simulink model "sampleModel240"  (R2021b)
settings: Solver=VariableStepAuto  StartTime=0.0  StopTime=10.0  RelTol=1e-3
undefined symbols (not defined in the file or in its folder): DiscIntNeverNeededParam, Newton, Raphson
libraries: simulink x11, slpidlib x4
settings Model: Creator=user  LastModifiedBy=user

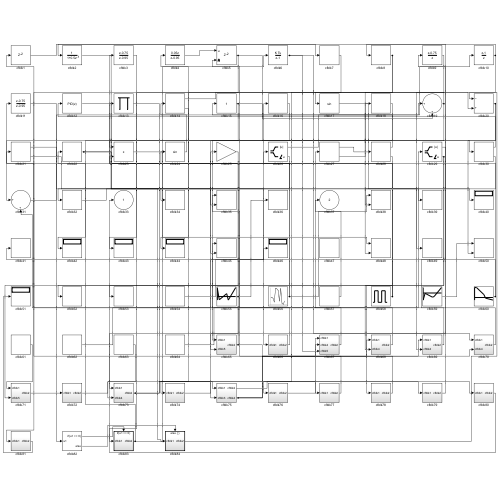
[thumbnail: Simulink's stored preview of the top-level diagram]
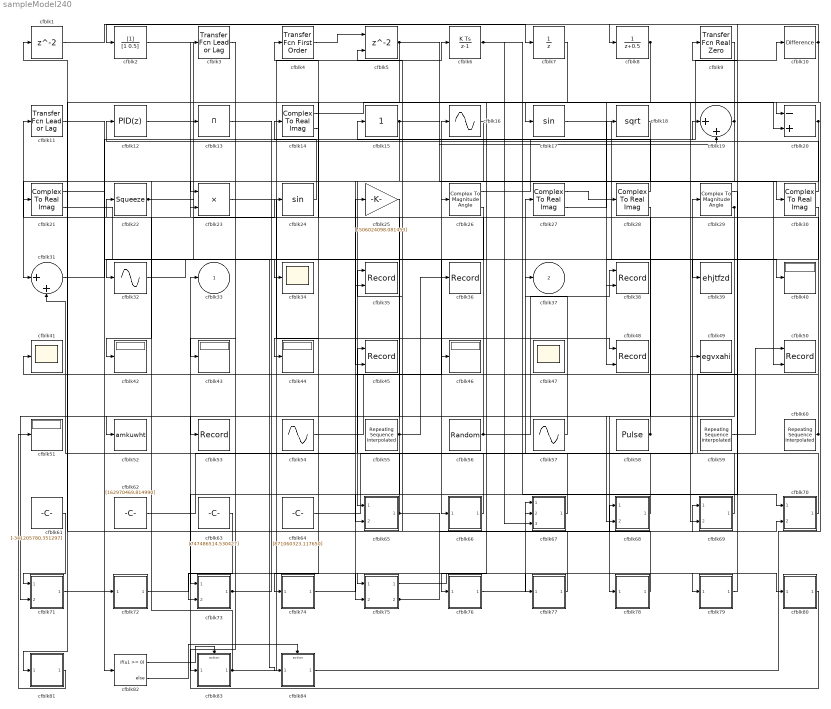
== system sampleModel240 ==
  cfblk1 : Delay  SampleTime=1
  cfblk10 : simulink/Discrete/Difference  ICPrevInput=0.0  OutMin=[]  OutMax=[]  OutDataTypeStr=Inherit: Inherit via back propagation  OutDataType=fixdt(1, 16)  OutScaling=2^-10  DoSatur=off
  cfblk11 : simulink/Discrete/Transfer Fcn Lead or Lag  PoleZ=0.95  ZeroZ=0.75  ICPrevOutput=0.0  ICPrevInput=0.0  DoSatur=off
      settings: SourceProductBaseCode=SL
  cfblk12 : slpidlib/PID Controller  Controller=PID  Form=Parallel  TimeDomain=Discrete-time  UseExternalTs=off  SampleTime=1  IntegratorMethod=Forward Euler  FilterMethod=Forward Euler  ControllerParametersSource=internal  P=1  I=1  D=0  UseFilter=on  N=100  TunerSelectOption=Transfer Function Based (PID Tuner App)  InitialConditionSource=internal  InitialConditionForIntegrator=0  InitialConditionForFilter=0  DifferentiatorICPrevScaledInput=0  ExternalReset=none  TrackingMode=off  Kt=1  LimitOutput=off  SatLimitsSource=internal  UpperSaturationLimit=inf  LowerSaturationLimit=-inf  LinearizeAsGain=off  AntiWindupMode=none  Kb=1  POutMin=[]  POutMax=[]  IOutMin=[]  IOutMax=[]  DOutMin=[]  DOutMax=[]  NOutMin=[]  NOutMax=[]  SumOutMin=[]  SumOutMax=[]  SaturationOutMin=[]  SaturationOutMax=[]  PParamMin=[]  PParamMax=[]  IParamMin=[]  IParamMax=[]  DParamMin=[]  DParamMax=[]  NParamMin=[]  NParamMax=[]  KbParamMin=[]  KbParamMax=[]  KtParamMin=[]  KtParamMax=[]  KbOutMin=[]  KbOutMax=[]  KtOutMin=[]  KtOutMax=[]  IntegratorOutMin=[]  IntegratorOutMax=[]  FilterOutMin=[]  FilterOutMax=[]  SumI1OutMin=[]  SumI1OutMax=[]  SumI2OutMin=[]  SumI2OutMax=[]  SumI3OutMin=[]  SumI3OutMax=[]  SumI4OutMin=[]  SumI4OutMax=[]  SumDOutMin=[]  SumDOutMax=[]  DifferentiatorOutMin=[]  DifferentiatorOutMax=[]  FilterDiffOutCoefMin=[]  FilterDiffOutCoefMax=[]  ReciprocalOutMin=[]  ReciprocalOutMax=[]  SumDenOutMin=[]  SumDenOutMax=[]  SumNumOutMin=[]  SumNumOutMax=[]  DivideOutMin=[]  DivideOutMax=[]  UdiffTsProdOutMin=[]  UdiffTsProdOutMax=[]  NTsProdOutMin=[]  NTsProdOutMax=[]  UintegralTsProdOutMin=[]  UintegralTsProdOutMax=[]  UngainTsProdOutMin=[]  UngainTsProdOutMax=[]  IntegratorContinuousStateAttributes=''  IntegratorStateMustResolveToSignalObject=off  IntegratorRTWStateStorageClass=Auto  FilterContinuousStateAttributes=''  FilterStateMustResolveToSignalObject=off  FilterRTWStateStorageClass=Auto  ParallelPVariant=InternalParameters  IdealPVariant=Disabled  IVariant=InternalParameters  DVariant=InternalParameters  IntegratorVariant=Discrete  SatVariant=Disabled  AWVariant=Passthrough  PCopyVariant=Disabled  TRVariant=Disabled  FdbkBlocksVariant=Forward  IdealPFdbkVariant=Disabled  SatFdbkVariant=Disabled  DerivativeFilterVariant=ForwardEulerFilter  NVariant=InternalParameters  NCopyVariant=Disabled  FilterICVariant=InternalICsFilter  IntegratorICVariant=InternalICs  ExternalResetVariant=Disabled  TRSumVariant=Passthrough  SumFdbkVariant=Disabled  SumVariant=Sum_PID  TsampFilterVariant=InternalTs  TsampNgainVariant=Passthrough  TsampIntegralVariant=Passthrough  ExternalSaturationOutDataTypeStr=Inherit: Same as second input
  cfblk13 : Product  Inputs=*
  cfblk{14,21,27..28,30} (5 alike) : ComplexToRealImag
  cfblk15 : simulink/Math Operations/Slider Gain  gain=1  low=0  high=2
  cfblk16 : Sin  TimeSource=Use external signal  SampleTime=0
  cfblk17 : Trigonometry
  cfblk18 : Sqrt  SaturateOnIntegerOverflow=on
  cfblk19 : Sum  Inputs=|++
  cfblk2 : DiscreteFilter  SampleTime=1
  cfblk20 : Sum  Inputs=-+
  cfblk22 : Squeeze
  cfblk23 : Product  Inputs=**
  cfblk24 : Trigonometry
  cfblk25 : Gain  Gain=[-506024098.081453]
  cfblk26 : ComplexToMagnitudeAngle
  cfblk29 : ComplexToMagnitudeAngle
  cfblk3 : simulink/Discrete/Transfer Fcn Lead or Lag  PoleZ=0.95  ZeroZ=0.75  ICPrevOutput=0.0  ICPrevInput=0.0  DoSatur=off
      settings: SourceProductBaseCode=SL
  cfblk31 : Sum  Inputs=|++
  cfblk32 : Sin  TimeSource=Use external signal  SampleTime=0
  cfblk34 : Scope
  cfblk35 : Record  FileSettingsInternal="{\"entries\":[{\"content\":{\"excelSettings\":{\"content\":{},\"type\":\"Streamout.ExcelSettings\"}},\"type\":\"Streamout.FileSettingStorage\",\"uuid\":\"784594ac-7453-4d0e-99dc-230d746005aa\"}],\"packageUris\":[\"http://schema.mathworks.com/mf0/streamout_blocks/R2020a\"],\"version\":\"1.0\"}"  Layout=[1 1]  SignalsInternal="{\"entries\":[{\"content\":{\"signals\":[{\"content\":{\"blockPath\":[\"sampleModel240/cfblk35\"],\"channel\":[],\"dimensions\":[1],\"domain\":\"sampleModel240/cfblk35\",\"lineColor\":\"#a2142f\",\"plots\":[1],\"port\":1,\"sid\":[\"\"],\"signalID\":9509,\"signalName\":\"cfblk78\"},\"type\":\"RecordBlkView.Signal\",\"uuid\":\"67d133b5-3512-448e-9778-6e57d9e23972\"},{\"content\":{\"blockPath\":[\"sampleModel240/cfblk35\"],\"channel\":[],\"dimensions\":[1],\"domain\":\"sampleModel240/cfblk35\",\"lineColor\":\"#139fff\",\"plots\":[1],\"port\":2,\"sid\":[\"\"],\"signalID\":9513,\"signalName\":\"cfblk11\"},\"type\":\"RecordBlkView.Signal\",\"uuid\":\"cb733c9c-883c-4945-886a-7784a95311ae\"}]},\"type\":\"RecordBlkView.InputSignals\",\"uuid\":\"c81b2700-d0a8-42b7-850e-26af2fe65ad5\"}],\"packageUris\":[\"http://schema.mathworks.com/mf0/streamout_blocks/R2020a\"],\"version\":\"1.0\"}"  VisualizationBindings="{\"xyplotplugin\":{\"info\":[{\"series\":[{\"bindingParametersList\":[{\"parameter\":\"X-Axis\",\"signalID\":9509,\"signalName\":\"cfblk78\"},{\"parameter\":\"Y-Axis\",\"signalID\":9513,\"signalName\":\"cfblk11\"}],\"seriesID\":32095}],\"subplotID\":1}]}}"  CompatibilityTag=XY
  cfblk36 : Record  FileSettingsInternal="{\"entries\":[{\"content\":{\"excelSettings\":{\"content\":{},\"type\":\"Streamout.ExcelSettings\"}},\"type\":\"Streamout.FileSettingStorage\",\"uuid\":\"b1a04026-dae7-46c6-8295-c1d018ed7cb2\"}],\"packageUris\":[\"http://schema.mathworks.com/mf0/streamout_blocks/R2020a\"],\"version\":\"1.0\"}"  SignalsInternal="{\"entries\":[{\"content\":{\"signals\":[{\"content\":{\"blockPath\":[\"sampleModel240/cfblk36\"],\"channel\":[],\"dimensions\":[1],\"domain\":\"sampleModel240/cfblk36\",\"lineColor\":\"#fe330a\",\"plots\":[1],\"port\":1,\"sid\":[\"\"],\"signalID\":9517,\"signalName\":\"cfblk55\"},\"type\":\"RecordBlkView.Signal\",\"uuid\":\"e81319b0-4fc9-46b2-b889-44dd591dc2c1\"}]},\"type\":\"RecordBlkView.InputSignals\",\"uuid\":\"d2d26a79-a2f7-4346-9dc2-1209bdb2fd03\"}],\"packageUris\":[\"http://schema.mathworks.com/mf0/streamout_blocks/R2020a\"],\"version\":\"1.0\"}"  VisualizationBindings="{\"sparklinesplugin\":{\"info\":[{\"bindingParametersList\":[],\"subplotID\":1}]}}"
  cfblk38 : Record  FileSettingsInternal="{\"entries\":[{\"content\":{\"excelSettings\":{\"content\":{},\"type\":\"Streamout.ExcelSettings\"}},\"type\":\"Streamout.FileSettingStorage\",\"uuid\":\"2b43e5d5-5da2-4669-81f9-69979c1bbe93\"}],\"packageUris\":[\"http://schema.mathworks.com/mf0/streamout_blocks/R2020a\"],\"version\":\"1.0\"}"  Layout=[1 1]  SignalsInternal="{\"entries\":[{\"content\":{\"signals\":[{\"content\":{\"blockPath\":[\"sampleModel240/cfblk38\"],\"channel\":[],\"dimensions\":[1],\"domain\":\"sampleModel240/cfblk38\",\"lineColor\":\"#a2142f\",\"plots\":[1],\"port\":1,\"sid\":[\"\"],\"signalID\":9521,\"signalName\":\"cfblk56\"},\"type\":\"RecordBlkView.Signal\",\"uuid\":\"72868b1f-4b0c-4be8-a2f7-40a7ef09af74\"},{\"content\":{\"blockPath\":[\"sampleModel240/cfblk38\"],\"channel\":[],\"dimensions\":[1],\"domain\":\"sampleModel240/cfblk38\",\"lineColor\":\"#139fff\",\"plots\":[1],\"port\":2,\"sid\":[\"\"],\"signalID\":9525,\"signalName\":\"cfblk30:2\"},\"type\":\"RecordBlkView.Signal\",\"uuid\":\"c76db0be-58e1-43fe-a83a-5ac3cfeabec3\"}]},\"type\":\"RecordBlkView.InputSignals\",\"uuid\":\"6d449aed-7e25-487a-9f87-ca08451d6c3a\"}],\"packageUris\":[\"http://schema.mathworks.com/mf0/streamout_blocks/R2020a\"],\"version\":\"1.0\"}"  VisualizationBindings="{\"xyplotplugin\":{\"info\":[{\"series\":[{\"bindingParametersList\":[{\"parameter\":\"X-Axis\",\"signalID\":9521,\"signalName\":\"cfblk56\"},{\"parameter\":\"Y-Axis\",\"signalID\":9525,\"signalName\":\"cfblk30:2\"}],\"seriesID\":59541}],\"subplotID\":1}]}}"  CompatibilityTag=XY
  cfblk39 : ToWorkspace  VariableName=ehjtfzd  SaveFormat=Timeseries  SampleTime=-1
  cfblk4 : simulink/Discrete/Transfer Fcn First Order  PoleZ=0.95  ICPrevOutput=0.0  DoSatur=off
  cfblk{40,42..44,46,51} (6 alike) : Display
  cfblk41 : Scope
  cfblk45 : Record  FileSettingsInternal="{\"entries\":[{\"content\":{\"excelSettings\":{\"content\":{},\"type\":\"Streamout.ExcelSettings\"}},\"type\":\"Streamout.FileSettingStorage\",\"uuid\":\"011ed913-79cb-4d04-904d-059d5477b360\"}],\"packageUris\":[\"http://schema.mathworks.com/mf0/streamout_blocks/R2020a\"],\"version\":\"1.0\"}"  Layout=[1 1]  SignalsInternal="{\"entries\":[{\"content\":{\"signals\":[{\"content\":{\"blockPath\":[\"sampleModel240/cfblk45\"],\"channel\":[],\"dimensions\":[1],\"domain\":\"sampleModel240/cfblk45\",\"lineColor\":\"#a2142f\",\"plots\":[1],\"port\":1,\"sid\":[\"\"],\"signalID\":9529,\"signalName\":\"cfblk67\"},\"type\":\"RecordBlkView.Signal\",\"uuid\":\"2900f96a-5edd-414d-b1fc-4191916f856c\"},{\"content\":{\"blockPath\":[\"sampleModel240/cfblk45\"],\"channel\":[],\"dimensions\":[1],\"domain\":\"sampleModel240/cfblk45\",\"lineColor\":\"#139fff\",\"plots\":[1],\"port\":2,\"sid\":[\"\"],\"signalID\":9533,\"signalName\":\"cfblk18\"},\"type\":\"RecordBlkView.Signal\",\"uuid\":\"83d649fc-fadd-439a-a8a7-d41cb33b9e8b\"}]},\"type\":\"RecordBlkView.InputSignals\",\"uuid\":\"9494aa0c-8dd6-4fcb-9a53-fd06893e11f2\"}],\"packageUris\":[\"http://schema.mathworks.com/mf0/streamout_blocks/R2020a\"],\"version\":\"1.0\"}"  VisualizationBindings="{\"xyplotplugin\":{\"info\":[{\"series\":[{\"bindingParametersList\":[{\"parameter\":\"X-Axis\",\"signalID\":9529,\"signalName\":\"cfblk67\"},{\"parameter\":\"Y-Axis\",\"signalID\":9533,\"signalName\":\"cfblk18\"}],\"seriesID\":51705}],\"subplotID\":1}]}}"  CompatibilityTag=XY
  cfblk47 : Scope
      settings: Floating=on
  cfblk48 : Record  FileSettingsInternal="{\"entries\":[{\"content\":{\"excelSettings\":{\"content\":{},\"type\":\"Streamout.ExcelSettings\"}},\"type\":\"Streamout.FileSettingStorage\",\"uuid\":\"3f33d199-868f-4f88-8702-0c4e5cfbf297\"}],\"packageUris\":[\"http://schema.mathworks.com/mf0/streamout_blocks/R2020a\"],\"version\":\"1.0\"}"  Layout=[1 1]  SignalsInternal="{\"entries\":[{\"content\":{\"signals\":[{\"content\":{\"blockPath\":[\"sampleModel240/cfblk48\"],\"channel\":[],\"dimensions\":[1],\"domain\":\"sampleModel240/cfblk48\",\"lineColor\":\"#a2142f\",\"plots\":[1],\"port\":1,\"sid\":[\"\"],\"signalID\":9537,\"signalName\":\"cfblk23\"},\"type\":\"RecordBlkView.Signal\",\"uuid\":\"ef2c7adb-1fb0-4c30-94cd-a61b1754e238\"},{\"content\":{\"blockPath\":[\"sampleModel240/cfblk48\"],\"channel\":[],\"dimensions\":[1],\"domain\":\"sampleModel240/cfblk48\",\"lineColor\":\"#139fff\",\"plots\":[1],\"port\":2,\"sid\":[\"\"],\"signalID\":9541,\"signalName\":\"cfblk8\"},\"type\":\"RecordBlkView.Signal\",\"uuid\":\"7ee245d3-5c2c-4c0d-a9a7-1766b601d128\"}]},\"type\":\"RecordBlkView.InputSignals\",\"uuid\":\"d6d367e3-47e7-4bb5-8610-e507c1deec50\"}],\"packageUris\":[\"http://schema.mathworks.com/mf0/streamout_blocks/R2020a\"],\"version\":\"1.0\"}"  VisualizationBindings="{\"xyplotplugin\":{\"info\":[{\"series\":[{\"bindingParametersList\":[{\"parameter\":\"X-Axis\",\"signalID\":9537,\"signalName\":\"cfblk23\"},{\"parameter\":\"Y-Axis\",\"signalID\":9541,\"signalName\":\"cfblk8\"}],\"seriesID\":9547}],\"subplotID\":1}]}}"  CompatibilityTag=XY
  cfblk49 : ToWorkspace  VariableName=egvxahi  SaveFormat=Timeseries  SampleTime=-1
  cfblk5 : Delay  ShowEnablePort=on  SampleTime=1
      settings: InputPortMap=u0,e6
  cfblk50 : Record  FileSettingsInternal="{\"entries\":[{\"content\":{\"excelSettings\":{\"content\":{},\"type\":\"Streamout.ExcelSettings\"}},\"type\":\"Streamout.FileSettingStorage\",\"uuid\":\"a7323de5-4913-44b3-ba6b-b7b4a20015af\"}],\"packageUris\":[\"http://schema.mathworks.com/mf0/streamout_blocks/R2020a\"],\"version\":\"1.0\"}"  Layout=[1 1]  SignalsInternal="{\"entries\":[{\"content\":{\"signals\":[{\"content\":{\"blockPath\":[\"sampleModel240/cfblk50\"],\"channel\":[],\"dimensions\":[1],\"domain\":\"sampleModel240/cfblk50\",\"lineColor\":\"#a2142f\",\"plots\":[1],\"port\":1,\"sid\":[\"\"],\"signalID\":9545,\"signalName\":\"cfblk59\"},\"type\":\"RecordBlkView.Signal\",\"uuid\":\"c6728527-33a3-402b-b809-e9ba282c6234\"},{\"content\":{\"blockPath\":[\"sampleModel240/cfblk50\"],\"channel\":[],\"dimensions\":[1],\"domain\":\"sampleModel240/cfblk50\",\"lineColor\":\"#139fff\",\"plots\":[1],\"port\":2,\"sid\":[\"\"],\"signalID\":9549,\"signalName\":\"cfblk20\"},\"type\":\"RecordBlkView.Signal\",\"uuid\":\"f80126da-2248-4c76-bb2b-053e64c3d372\"}]},\"type\":\"RecordBlkView.InputSignals\",\"uuid\":\"537812bb-574c-401c-a38e-823000144505\"}],\"packageUris\":[\"http://schema.mathworks.com/mf0/streamout_blocks/R2020a\"],\"version\":\"1.0\"}"  VisualizationBindings="{\"xyplotplugin\":{\"info\":[{\"series\":[{\"bindingParametersList\":[{\"parameter\":\"X-Axis\",\"signalID\":9545,\"signalName\":\"cfblk59\"},{\"parameter\":\"Y-Axis\",\"signalID\":9549,\"signalName\":\"cfblk20\"}],\"seriesID\":24204}],\"subplotID\":1}]}}"  CompatibilityTag=XY
  cfblk52 : ToWorkspace  VariableName=amkuwht  SaveFormat=Timeseries  SampleTime=-1
  cfblk53 : Record  FileSettingsInternal="{\"entries\":[{\"content\":{\"excelSettings\":{\"content\":{},\"type\":\"Streamout.ExcelSettings\"}},\"type\":\"Streamout.FileSettingStorage\",\"uuid\":\"062d2fcb-1db7-4794-8512-aa17b3a50389\"}],\"packageUris\":[\"http://schema.mathworks.com/mf0/streamout_blocks/R2020a\"],\"version\":\"1.0\"}"  SignalsInternal="{\"entries\":[{\"content\":{\"signals\":[{\"content\":{\"blockPath\":[\"sampleModel240/cfblk53\"],\"channel\":[],\"dimensions\":[1],\"domain\":\"sampleModel240/cfblk53\",\"lineColor\":\"#139fff\",\"plots\":[1],\"port\":1,\"sid\":[\"\"],\"signalID\":9553,\"signalName\":\"cfblk5\"},\"type\":\"RecordBlkView.Signal\",\"uuid\":\"004bb81a-6ea3-4587-b6bd-6712f3703243\"}]},\"type\":\"RecordBlkView.InputSignals\",\"uuid\":\"4f08d72a-b7cb-43bf-9134-c95f940a5c70\"}],\"packageUris\":[\"http://schema.mathworks.com/mf0/streamout_blocks/R2020a\"],\"version\":\"1.0\"}"  VisualizationBindings="{\"sparklinesplugin\":{\"info\":[{\"bindingParametersList\":[],\"subplotID\":1}]}}"
  cfblk54 : Sin  Amplitude=[927282513.188277]  Bias=[-745493718.771142]  SampleTime=0
  cfblk55 : simulink/Sources/Repeating Sequence Interpolated  OutValues=[757544215.990310, -282071434.589029, 262873848.324371, -311269752.017773, 843048073.550432]  TimeValues=[0 0.1 0.5 0.6 1].'  LookUpMeth=Use Input Nearest  tsamp=0.01  OutMin=[]  OutMax=[]  OutDataTypeStr=double  OutputDataTypeScalingMode=double  OutDataType=fixdt(0,8)  OutScaling=2^-10
  cfblk56 : RandomNumber  Mean=[-10045.091864]  Variance=[72480.359942]  Seed=[426711266.000000]  SampleTime=0.1
  cfblk57 : Sin  Amplitude=[314477199.179577]  Bias=[-113427137.959207]  SampleTime=0
  cfblk58 : DiscretePulseGenerator  PulseType=Time based  Amplitude=[121664850.347592]  Period=[59251250.117236]  PulseWidth=5  PhaseDelay=[3.000000]
  cfblk59 : simulink/Sources/Repeating Sequence Interpolated  OutValues=[-995730294.606779, -23875285.976552, -567680596.972897, -484368832.556859, 819766545.228171]  TimeValues=[0 0.1 0.5 0.6 1].'  LookUpMeth=Use Input Above  tsamp=0.01  OutMin=[]  OutMax=[]  OutDataTypeStr=double  OutputDataTypeScalingMode=double  OutDataType=fixdt(0,8)  OutScaling=2^-10
  cfblk6 : DiscreteIntegrator  ICPrevOutput=DiscIntNeverNeededParam  ICPrevScaledInput=DiscIntNeverNeededParam
  cfblk60 : simulink/Sources/Repeating Sequence Interpolated  OutValues=[884652968.497208, 878168725.746222, 262963678.617603, -60188493.029042, -217965531.630262]  TimeValues=[0 0.1 0.5 0.6 1].'  LookUpMeth=Use Input Nearest  tsamp=0.01  OutMin=[]  OutMax=[]  OutDataTypeStr=double  OutputDataTypeScalingMode=double  OutDataType=fixdt(0,8)  OutScaling=2^-10
  cfblk61 : Constant  Value=[-341205780.351297]  SampleTime=1
  cfblk62 : Constant  Value=[162970469.814990]  SampleTime=1
  cfblk63 : Constant  Value=[747486514.530427]  SampleTime=1
  cfblk64 : Constant  Value=[871060323.117650]  SampleTime=1
  cfblk65 : Subsystem
  cfblk66 : Subsystem
  cfblk67 : Subsystem
  cfblk68 : Subsystem
  cfblk69 : Subsystem
  cfblk7 : UnitDelay  HasFrameUpgradeWarning=on
  cfblk70 : Subsystem
  cfblk71 : Subsystem
  cfblk72 : Subsystem
  cfblk73 : Subsystem
  cfblk74 : Subsystem
  cfblk75 : Subsystem
  cfblk76 : Subsystem
  cfblk77 : Subsystem
  cfblk78 : Subsystem
  cfblk79 : Subsystem
  cfblk8 : DiscreteTransferFcn  SampleTime=1
  cfblk80 : Subsystem
  cfblk81 : Subsystem
  cfblk82 : If  IfExpression=u1 >= 0  SampleTime=1
  cfblk83 : Subsystem  TreatAsAtomicUnit=on
  cfblk84 : Subsystem  TreatAsAtomicUnit=on
  cfblk9 : simulink/Discrete/Transfer Fcn Real Zero  ZeroZ=0.75  ICPrevInput=0.0  DoSatur=off
      settings: SourceProductBaseCode=SL
  cfblk33 : Outport
  cfblk37 : Outport  Port=2
  wires:
  cfblk58/1 -> cfblk11/1, cfblk52/1, cfblk23/2
  cfblk83/1(cfblk2) -> cfblk6/1, cfblk22/1
  cfblk64/1 -> cfblk29/1
  cfblk75/1(cfblk2) -> cfblk79/1(cfblk1)
  cfblk59/1 -> cfblk50/1
  cfblk24/1 -> cfblk14/1
  cfblk80/1(cfblk2) -> cfblk33/1
  cfblk8/1 -> cfblk74/1(cfblk1), cfblk48/2
  cfblk15/1 -> cfblk31/1, cfblk30/1
  cfblk79/1(cfblk2) -> cfblk2/1
  cfblk26/1 -> cfblk10/1
  cfblk32/1 -> cfblk84/1(cfblk1)
  cfblk16/1 -> cfblk65/1(cfblk1)
  cfblk67/1(cfblk2) -> cfblk45/1
  cfblk1/1 -> cfblk7/1
  cfblk26/2 -> cfblk32/1
  cfblk17/1 -> cfblk39/1
  cfblk18/1 -> cfblk45/2
  cfblk29/1 -> cfblk65/2(cfblk5)
  cfblk27/1 -> cfblk28/1
  cfblk54/1 -> cfblk16/1
  cfblk12/1 -> cfblk66/1(cfblk1)
  cfblk4/1 -> cfblk5/1
  cfblk70/1(cfblk2) -> cfblk9/1
  cfblk61/1 -> cfblk71/1(cfblk1)
  cfblk10/1 -> cfblk8/1, cfblk69/2(cfblk4)
  cfblk60/1 -> cfblk41/1, cfblk13/1
  cfblk55/1 -> cfblk73/1(cfblk1), cfblk3/1, cfblk36/1
  cfblk2/1 -> cfblk40/1
  cfblk20/1 -> cfblk42/1, cfblk50/2
  cfblk27/2 -> cfblk18/1
  cfblk69/1(cfblk2) -> cfblk5/2
  cfblk23/1 -> cfblk48/1
  cfblk62/1 -> cfblk25/1
  cfblk6/1 -> cfblk70/1(cfblk1), cfblk67/3(cfblk5)
  cfblk5/1 -> cfblk53/1, cfblk19/2
  cfblk7/1 -> cfblk81/1(cfblk1)
  cfblk63/1 -> cfblk73/2(cfblk4)
  cfblk68/1(cfblk2) -> cfblk27/1
  cfblk9/1 -> cfblk76/1(cfblk1)
  cfblk84/1(cfblk2) -> cfblk20/1
  cfblk22/1 -> cfblk34/1, cfblk24/1
  cfblk28/1 -> cfblk15/1
  cfblk19/1 -> cfblk17/1, cfblk23/1
  cfblk73/1(cfblk2) -> cfblk75/1(cfblk1), cfblk77/1(cfblk1)
  cfblk3/1 -> cfblk43/1
  cfblk56/1 -> cfblk38/1, cfblk26/1, cfblk4/1
  cfblk21/1 -> cfblk82/1
  cfblk30/1 -> cfblk12/1
  cfblk78/1(cfblk2) -> cfblk35/1
  cfblk57/1 -> cfblk37/1
  cfblk21/2 -> cfblk49/1
  cfblk31/1 -> cfblk19/1
  cfblk30/2 -> cfblk38/2
  cfblk71/1(cfblk2) -> cfblk72/1(cfblk1)
  cfblk66/1(cfblk2) -> cfblk31/2
  cfblk25/1 -> cfblk83/1(cfblk1)
  cfblk81/1(cfblk2) -> cfblk51/1
  cfblk28/2 -> cfblk71/2(cfblk5)
  cfblk14/1 -> cfblk20/2
  cfblk13/1 -> cfblk75/2(cfblk3)
  cfblk65/1(cfblk2) -> cfblk1/1, cfblk70/2(cfblk4)
  cfblk29/2 -> cfblk78/1(cfblk1), cfblk68/2(cfblk4)
  cfblk11/1 -> cfblk35/2
  cfblk72/1(cfblk2) -> cfblk80/1(cfblk1)
  cfblk14/2 -> cfblk44/1
  cfblk74/1(cfblk2) -> cfblk46/1
  cfblk77/1(cfblk2) -> cfblk21/1
  cfblk75/2(cfblk4) -> cfblk68/1(cfblk1), cfblk69/1(cfblk1), cfblk67/2(cfblk4)
  cfblk76/1(cfblk2) -> cfblk67/1(cfblk1)
  cfblk82/1 -> cfblk83/Action
  cfblk82/2 -> cfblk84/Action

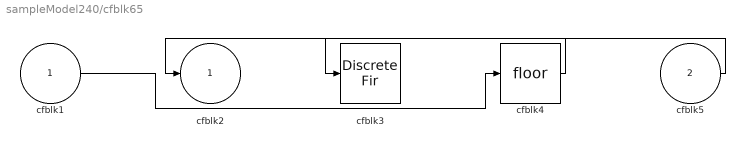
== system sampleModel240/cfblk65 ==
  cfblk1 : Inport
  cfblk5 : Inport  Port=2
  cfblk3 : DiscreteFir  SampleTime=1
  cfblk4 : Rounding
  cfblk2 : Outport
  wires:
  cfblk4/1 -> cfblk2/1
  cfblk1/1 -> cfblk4/1
  cfblk5/1 -> cfblk3/1

== system sampleModel240/cfblk66 ==
  cfblk1 : Inport
  cfblk3 : simulink/Discrete/Transfer Fcn Lead or Lag  PoleZ=0.95  ZeroZ=0.75  ICPrevOutput=0.0  ICPrevInput=0.0  DoSatur=off
      settings: SourceProductBaseCode=SL
  cfblk2 : Outport
  wires:
  cfblk3/1 -> cfblk2/1
  cfblk1/1 -> cfblk3/1

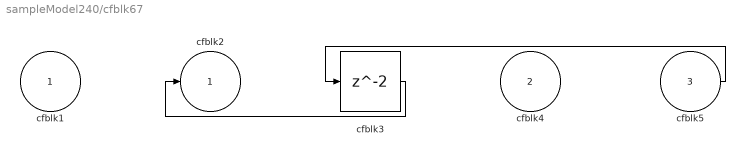
== system sampleModel240/cfblk67 ==
  cfblk1 : Inport
  cfblk4 : Inport  Port=2
  cfblk5 : Inport  Port=3
  cfblk3 : Delay  SampleTime=1
  cfblk2 : Outport
  wires:
  cfblk5/1 -> cfblk3/1
  cfblk3/1 -> cfblk2/1

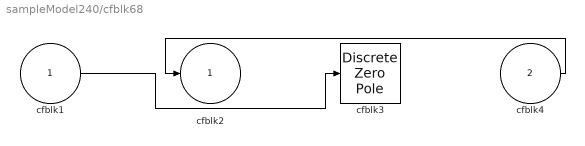
== system sampleModel240/cfblk68 ==
  cfblk1 : Inport
  cfblk4 : Inport  Port=2
  cfblk3 : DiscreteZeroPole  Poles=[0 0.5]  Gain=1
  cfblk2 : Outport
  wires:
  cfblk4/1 -> cfblk2/1
  cfblk1/1 -> cfblk3/1

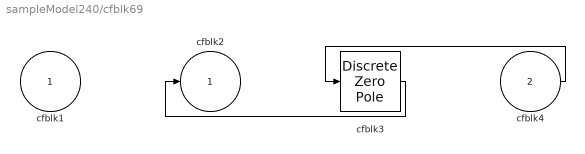
== system sampleModel240/cfblk69 ==
  cfblk1 : Inport
  cfblk4 : Inport  Port=2
  cfblk3 : DiscreteZeroPole  Poles=[0 0.5]  Gain=1
  cfblk2 : Outport
  wires:
  cfblk4/1 -> cfblk3/1
  cfblk3/1 -> cfblk2/1

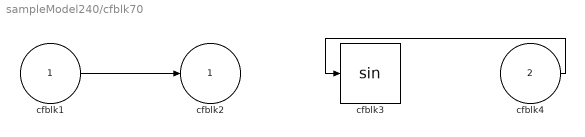
== system sampleModel240/cfblk70 ==
  cfblk1 : Inport
  cfblk4 : Inport  Port=2
  cfblk3 : Trigonometry
  cfblk2 : Outport
  wires:
  cfblk4/1 -> cfblk3/1
  cfblk1/1 -> cfblk2/1

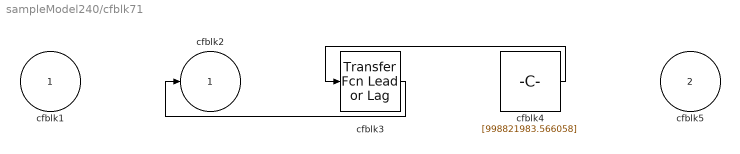
== system sampleModel240/cfblk71 ==
  cfblk1 : Inport
  cfblk5 : Inport  Port=2
  cfblk3 : simulink/Discrete/Transfer Fcn Lead or Lag  PoleZ=0.95  ZeroZ=0.75  ICPrevOutput=0.0  ICPrevInput=0.0  DoSatur=off
      settings: SourceProductBaseCode=SL
  cfblk4 : Constant  Value=[998821983.566058]  SampleTime=1
  cfblk2 : Outport
  wires:
  cfblk4/1 -> cfblk3/1
  cfblk3/1 -> cfblk2/1

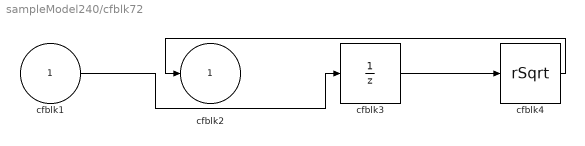
== system sampleModel240/cfblk72 ==
  cfblk1 : Inport
  cfblk3 : UnitDelay  HasFrameUpgradeWarning=on
  cfblk4 : Sqrt  Operator=rSqrt  AlgorithmType=Newton-Raphson  SaturateOnIntegerOverflow=on
  cfblk2 : Outport
  wires:
  cfblk4/1 -> cfblk2/1
  cfblk1/1 -> cfblk3/1
  cfblk3/1 -> cfblk4/1

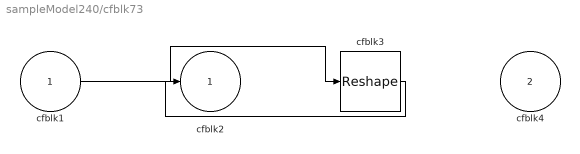
== system sampleModel240/cfblk73 ==
  cfblk1 : Inport
  cfblk4 : Inport  Port=2
  cfblk3 : Reshape
  cfblk2 : Outport
  wires:
  cfblk1/1 -> cfblk3/1
  cfblk3/1 -> cfblk2/1

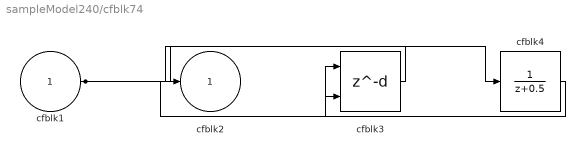
== system sampleModel240/cfblk74 ==
  cfblk1 : Inport
  cfblk3 : Delay  DelayLengthSource=Input port  SampleTime=1
      settings: InputPortMap=u0,p1
  cfblk4 : DiscreteTransferFcn  SampleTime=1
  cfblk2 : Outport
  wires:
  cfblk1/1 -> cfblk4/1, cfblk3/2
  cfblk4/1 -> cfblk3/1
  cfblk3/1 -> cfblk2/1

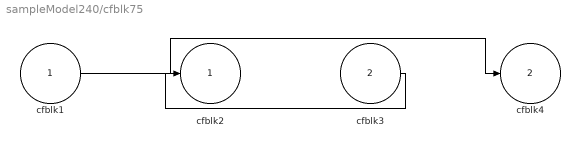
== system sampleModel240/cfblk75 ==
  cfblk1 : Inport
  cfblk3 : Inport  Port=2
  cfblk2 : Outport
  cfblk4 : Outport  Port=2
  wires:
  cfblk1/1 -> cfblk4/1
  cfblk3/1 -> cfblk2/1

== system sampleModel240/cfblk76 ==
  cfblk1 : Inport
  cfblk3 : Product  Inputs=**
  cfblk2 : Outport
  wires:
  cfblk1/1 -> cfblk3/1, cfblk3/2
  cfblk3/1 -> cfblk2/1

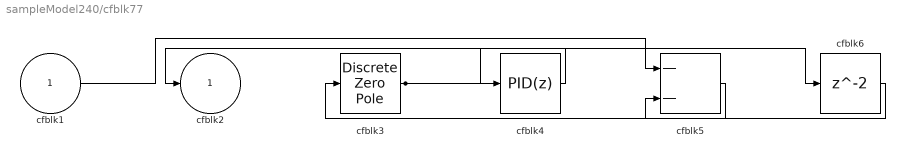
== system sampleModel240/cfblk77 ==
  cfblk1 : Inport
  cfblk3 : DiscreteZeroPole  Poles=[0 0.5]  Gain=1
  cfblk4 : slpidlib/PID Controller  Controller=PID  Form=Parallel  TimeDomain=Discrete-time  UseExternalTs=off  SampleTime=1  IntegratorMethod=Forward Euler  FilterMethod=Forward Euler  ControllerParametersSource=internal  P=1  I=1  D=0  UseFilter=on  N=100  TunerSelectOption=Transfer Function Based (PID Tuner App)  InitialConditionSource=internal  InitialConditionForIntegrator=0  InitialConditionForFilter=0  DifferentiatorICPrevScaledInput=0  ExternalReset=none  TrackingMode=off  Kt=1  LimitOutput=off  SatLimitsSource=internal  UpperSaturationLimit=inf  LowerSaturationLimit=-inf  LinearizeAsGain=off  AntiWindupMode=none  Kb=1  POutMin=[]  POutMax=[]  IOutMin=[]  IOutMax=[]  DOutMin=[]  DOutMax=[]  NOutMin=[]  NOutMax=[]  SumOutMin=[]  SumOutMax=[]  SaturationOutMin=[]  SaturationOutMax=[]  PParamMin=[]  PParamMax=[]  IParamMin=[]  IParamMax=[]  DParamMin=[]  DParamMax=[]  NParamMin=[]  NParamMax=[]  KbParamMin=[]  KbParamMax=[]  KtParamMin=[]  KtParamMax=[]  KbOutMin=[]  KbOutMax=[]  KtOutMin=[]  KtOutMax=[]  IntegratorOutMin=[]  IntegratorOutMax=[]  FilterOutMin=[]  FilterOutMax=[]  SumI1OutMin=[]  SumI1OutMax=[]  SumI2OutMin=[]  SumI2OutMax=[]  SumI3OutMin=[]  SumI3OutMax=[]  SumI4OutMin=[]  SumI4OutMax=[]  SumDOutMin=[]  SumDOutMax=[]  DifferentiatorOutMin=[]  DifferentiatorOutMax=[]  FilterDiffOutCoefMin=[]  FilterDiffOutCoefMax=[]  ReciprocalOutMin=[]  ReciprocalOutMax=[]  SumDenOutMin=[]  SumDenOutMax=[]  SumNumOutMin=[]  SumNumOutMax=[]  DivideOutMin=[]  DivideOutMax=[]  UdiffTsProdOutMin=[]  UdiffTsProdOutMax=[]  NTsProdOutMin=[]  NTsProdOutMax=[]  UintegralTsProdOutMin=[]  UintegralTsProdOutMax=[]  UngainTsProdOutMin=[]  UngainTsProdOutMax=[]  IntegratorContinuousStateAttributes=''  IntegratorStateMustResolveToSignalObject=off  IntegratorRTWStateStorageClass=Auto  FilterContinuousStateAttributes=''  FilterStateMustResolveToSignalObject=off  FilterRTWStateStorageClass=Auto  ParallelPVariant=InternalParameters  IdealPVariant=Disabled  IVariant=InternalParameters  DVariant=InternalParameters  IntegratorVariant=Discrete  SatVariant=Disabled  AWVariant=Passthrough  PCopyVariant=Disabled  TRVariant=Disabled  FdbkBlocksVariant=Forward  IdealPFdbkVariant=Disabled  SatFdbkVariant=Disabled  DerivativeFilterVariant=ForwardEulerFilter  NVariant=InternalParameters  NCopyVariant=Disabled  FilterICVariant=InternalICsFilter  IntegratorICVariant=InternalICs  ExternalResetVariant=Disabled  TRSumVariant=Passthrough  SumFdbkVariant=Disabled  SumVariant=Sum_PID  TsampFilterVariant=InternalTs  TsampNgainVariant=Passthrough  TsampIntegralVariant=Passthrough  ExternalSaturationOutDataTypeStr=Inherit: Same as second input
  cfblk5 : Sum  Inputs=--
  cfblk6 : Delay  SampleTime=1
  cfblk2 : Outport
  wires:
  cfblk4/1 -> cfblk2/1
  cfblk3/1 -> cfblk4/1, cfblk6/1
  cfblk1/1 -> cfblk5/1
  cfblk5/1 -> cfblk3/1
  cfblk6/1 -> cfblk5/2

== system sampleModel240/cfblk78 ==
  cfblk1 : Inport
  cfblk3 : DiscreteFir  SampleTime=1
  cfblk2 : Outport
  wires:
  cfblk1/1 -> cfblk2/1, cfblk3/1

== system sampleModel240/cfblk79 ==
  cfblk1 : Inport
  cfblk3 : Delay  DelayLengthSource=Input port  SampleTime=1
      settings: InputPortMap=u0,p1
  cfblk2 : Outport
  wires:
  cfblk1/1 -> cfblk2/1, cfblk3/1, cfblk3/2

== system sampleModel240/cfblk80 ==
  cfblk1 : Inport
  cfblk3 : slpidlib/PID Controller (2DOF)  Controller=PID  Form=Parallel  TimeDomain=Discrete-time  UseExternalTs=off  SampleTime=1  IntegratorMethod=Forward Euler  FilterMethod=Forward Euler  ControllerParametersSource=internal  P=1  I=1  D=0  UseFilter=on  N=100  b=1  c=1  TunerSelectOption=Transfer Function Based (PID Tuner App)  InitialConditionSource=internal  InitialConditionForIntegrator=0  InitialConditionForFilter=0  DifferentiatorICPrevScaledInput=0  ExternalReset=none  TrackingMode=off  Kt=1  LimitOutput=off  SatLimitsSource=internal  UpperSaturationLimit=inf  LowerSaturationLimit=-inf  LinearizeAsGain=off  AntiWindupMode=none  Kb=1  POutMin=[]  POutMax=[]  IOutMin=[]  IOutMax=[]  DOutMin=[]  DOutMax=[]  NOutMin=[]  NOutMax=[]  bOutMin=[]  bOutMax=[]  cOutMin=[]  cOutMax=[]  SumOutMin=[]  SumOutMax=[]  SaturationOutMin=[]  SaturationOutMax=[]  PParamMin=[]  PParamMax=[]  IParamMin=[]  IParamMax=[]  DParamMin=[]  DParamMax=[]  NParamMin=[]  NParamMax=[]  bParamMin=[]  bParamMax=[]  cParamMin=[]  cParamMax=[]  KbParamMin=[]  KbParamMax=[]  KtParamMin=[]  KtParamMax=[]  KbOutMin=[]  KbOutMax=[]  KtOutMin=[]  KtOutMax=[]  IntegratorOutMin=[]  IntegratorOutMax=[]  FilterOutMin=[]  FilterOutMax=[]  SumI1OutMin=[]  SumI1OutMax=[]  SumI2OutMin=[]  SumI2OutMax=[]  SumI3OutMin=[]  SumI3OutMax=[]  SumI4OutMin=[]  SumI4OutMax=[]  SumDOutMin=[]  SumDOutMax=[]  Sum1OutMin=[]  Sum1OutMax=[]  Sum2OutMin=[]  Sum2OutMax=[]  Sum3OutMin=[]  Sum3OutMax=[]  DifferentiatorOutMin=[]  DifferentiatorOutMax=[]  FilterDiffOutCoefMin=[]  FilterDiffOutCoefMax=[]  ReciprocalOutMin=[]  ReciprocalOutMax=[]  SumDenOutMin=[]  SumDenOutMax=[]  SumNumOutMin=[]  SumNumOutMax=[]  DivideOutMin=[]  DivideOutMax=[]  UdiffTsProdOutMin=[]  UdiffTsProdOutMax=[]  NTsProdOutMin=[]  NTsProdOutMax=[]  UintegralTsProdOutMin=[]  UintegralTsProdOutMax=[]  UngainTsProdOutMin=[]  UngainTsProdOutMax=[]  IntegratorContinuousStateAttributes=''  IntegratorStateMustResolveToSignalObject=off  IntegratorRTWStateStorageClass=Auto  FilterContinuousStateAttributes=''  FilterStateMustResolveToSignalObject=off  FilterRTWStateStorageClass=Auto  ParallelPVariant=InternalParameters  IdealPVariant=Disabled  IVariant=InternalParameters  DVariant=InternalParameters  bVariant=InternalParameters  cVariant=InternalParameters  IntegratorVariant=Discrete  SatVariant=Disabled  AWVariant=Passthrough  PCopyVariant=Disabled  TRVariant=Disabled  FdbkBlocksVariant=Forward  IdealPFdbkVariant=Disabled  SatFdbkVariant=Disabled  DerivativeFilterVariant=ForwardEulerFilter  NVariant=InternalParameters  NCopyVariant=Disabled  FilterICVariant=InternalICsFilter  IntegratorICVariant=InternalICs  ExternalResetVariant=Disabled  TRSumVariant=Passthrough  SumFdbkVariant=Disabled  SumVariant=Sum_PID  TsampFilterVariant=InternalTs  TsampNgainVariant=Passthrough  TsampIntegralVariant=Passthrough  ExternalSaturationOutDataTypeStr=Inherit: Same as second input
      settings: SourceProductBaseCode=SL
  cfblk2 : Outport
  wires:
  cfblk1/1 -> cfblk3/1, cfblk3/2
  cfblk3/1 -> cfblk2/1

== system sampleModel240/cfblk81 ==
  cfblk1 : Inport
  cfblk3 : Constant  Value=[-203881698.198706]  SampleTime=1
  cfblk2 : Outport
  wires:
  cfblk3/1 -> cfblk2/1

== system sampleModel240/cfblk83 ==
  cfblk1 : Inport
  Action Port : ActionPort  ActionPortLabel=if(u1 >= 0)
  cfblk3 : slpidlib/PID Controller  Controller=PID  Form=Parallel  TimeDomain=Discrete-time  UseExternalTs=off  SampleTime=-1  IntegratorMethod=Forward Euler  FilterMethod=Forward Euler  ControllerParametersSource=internal  P=1  I=1  D=0  UseFilter=on  N=100  TunerSelectOption=Transfer Function Based (PID Tuner App)  InitialConditionSource=internal  InitialConditionForIntegrator=0  InitialConditionForFilter=0  DifferentiatorICPrevScaledInput=0  ExternalReset=none  TrackingMode=off  Kt=1  LimitOutput=off  SatLimitsSource=internal  UpperSaturationLimit=inf  LowerSaturationLimit=-inf  LinearizeAsGain=off  AntiWindupMode=none  Kb=1  POutMin=[]  POutMax=[]  IOutMin=[]  IOutMax=[]  DOutMin=[]  DOutMax=[]  NOutMin=[]  NOutMax=[]  SumOutMin=[]  SumOutMax=[]  SaturationOutMin=[]  SaturationOutMax=[]  PParamMin=[]  PParamMax=[]  IParamMin=[]  IParamMax=[]  DParamMin=[]  DParamMax=[]  NParamMin=[]  NParamMax=[]  KbParamMin=[]  KbParamMax=[]  KtParamMin=[]  KtParamMax=[]  KbOutMin=[]  KbOutMax=[]  KtOutMin=[]  KtOutMax=[]  IntegratorOutMin=[]  IntegratorOutMax=[]  FilterOutMin=[]  FilterOutMax=[]  SumI1OutMin=[]  SumI1OutMax=[]  SumI2OutMin=[]  SumI2OutMax=[]  SumI3OutMin=[]  SumI3OutMax=[]  SumI4OutMin=[]  SumI4OutMax=[]  SumDOutMin=[]  SumDOutMax=[]  DifferentiatorOutMin=[]  DifferentiatorOutMax=[]  FilterDiffOutCoefMin=[]  FilterDiffOutCoefMax=[]  ReciprocalOutMin=[]  ReciprocalOutMax=[]  SumDenOutMin=[]  SumDenOutMax=[]  SumNumOutMin=[]  SumNumOutMax=[]  DivideOutMin=[]  DivideOutMax=[]  UdiffTsProdOutMin=[]  UdiffTsProdOutMax=[]  NTsProdOutMin=[]  NTsProdOutMax=[]  UintegralTsProdOutMin=[]  UintegralTsProdOutMax=[]  UngainTsProdOutMin=[]  UngainTsProdOutMax=[]  IntegratorContinuousStateAttributes=''  IntegratorStateMustResolveToSignalObject=off  IntegratorRTWStateStorageClass=Auto  FilterContinuousStateAttributes=''  FilterStateMustResolveToSignalObject=off  FilterRTWStateStorageClass=Auto  ParallelPVariant=InternalParameters  IdealPVariant=Disabled  IVariant=InternalParameters  DVariant=InternalParameters  IntegratorVariant=Discrete  SatVariant=Disabled  AWVariant=Passthrough  PCopyVariant=Disabled  TRVariant=Disabled  FdbkBlocksVariant=Forward  IdealPFdbkVariant=Disabled  SatFdbkVariant=Disabled  DerivativeFilterVariant=ForwardEulerFilter  NVariant=InternalParameters  NCopyVariant=Disabled  FilterICVariant=InternalICsFilter  IntegratorICVariant=InternalICs  ExternalResetVariant=Disabled  TRSumVariant=Passthrough  SumFdbkVariant=Disabled  SumVariant=Sum_PID  TsampFilterVariant=InternalTs  TsampNgainVariant=Passthrough  TsampIntegralVariant=Passthrough  ExternalSaturationOutDataTypeStr=Inherit: Same as second input
  cfblk2 : Outport
  wires:
  cfblk1/1 -> cfblk3/1
  cfblk3/1 -> cfblk2/1

== system sampleModel240/cfblk84 ==
  cfblk1 : Inport
  Action Port : ActionPort  ActionPortLabel=else
  cfblk3 : Sqrt  Operator=rSqrt  AlgorithmType=Newton-Raphson  SaturateOnIntegerOverflow=on
  cfblk2 : Outport
  wires:
  cfblk1/1 -> cfblk2/1, cfblk3/1
